simulink model "ur5_mb1"  (R2024b)
settings: Solver=VariableStepAuto  StartTime=0.0  StopTime=inf  RelTol=1e-3
values from neighbouring files (symbols this model uses):
  N = 500000    [te.m]
undefined symbols (not defined in the file or in its folder): X, Y, Z
libraries: sm_lib x89, nesl_utility x25, sldrtlib x1
(part 1 of 3)
settings Model: Creator=20844  LastModifiedBy=20844
settings ExplorerConfigSet: InternalSimMechanicsExplorerSettings="<ExplorerConfiguration><canonicalview>default</canonicalview><AnimationSetting><BasePlaybackSpeed>1.0</BasePlaybackSpeed><PlaybackSpeedFactor>1.0</PlaybackSpeedFactor></AnimationSetting><TilePanel><TileInfo><Tiles Columns=\"1\" Count=\"1\" Rows=\"1\"><Column Weight=\"1\"/><Row Weight=\"1\"/><Tile Height=\"1\" Width=\"1\" X=\"0\" Y=\"0\"/></Tiles></TileInfo><SceneInfo><SceneViewer><BGColor><R>0.60000002384185791</R><G>0.60000002384185791</G><B>0.60000002384185791</B></BGColor><Camera><DoPerspective>off</DoPerspective><Position><X>0.566882143907464497</X><Y>-0.926894596308694196</Y><Z>0.376591257371258314</Z></Position><Center><X>0.550100812264807226</X><Y>0.0723916711678013747</Y><Z>0.342748347608626824</Z></Center><Up><X>0.0212034026804047183</X><Y>0.0341957319134813531</Y><Z>0.999190205933622289</Z></Up><ViewLimDist>1</ViewLimDist><YLim>1.26913824826545474</YLim><XLim>1.85200174006144125</XLim></Camera></SceneViewer></SceneInfo></TilePanel><MechEditorPanel><Cameras/><GfxPanelCameraMap/><VideoCreator><PlaybackSpeedRatio>1.0</PlaybackSpeedRatio><FrameRate>30</FrameRate><VideoFormat>Motion JPEG AVI</VideoFormat><FrameSize>auto</FrameSize></VideoCreator></MechEditorPanel></ExplorerConfiguration>"

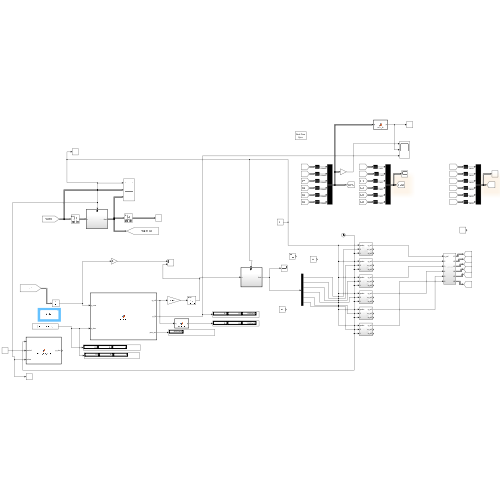
[thumbnail: Simulink's stored preview of the top-level diagram]
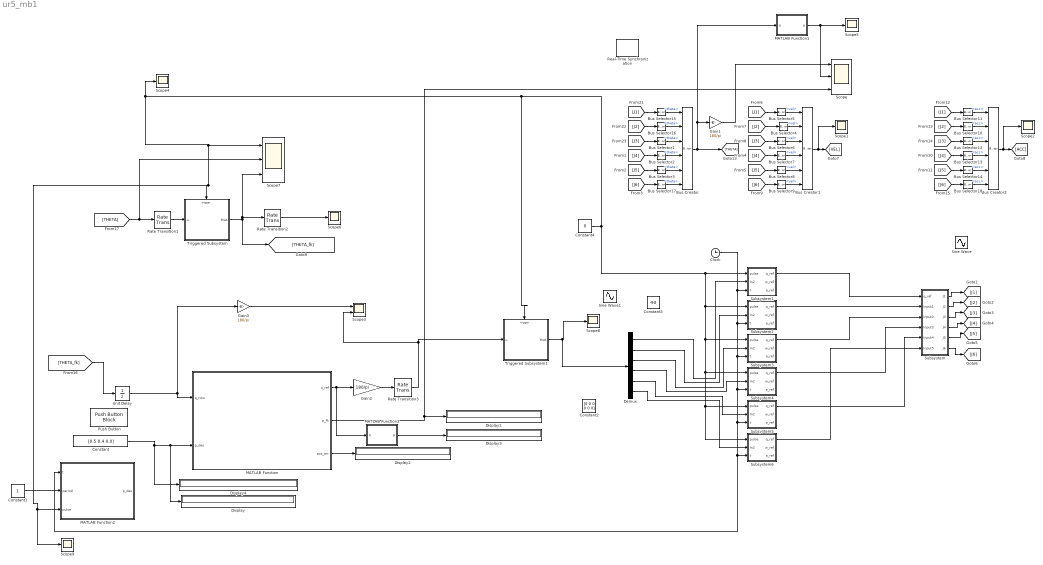
== system ur5_mb1 ==
  Bus Creator : BusCreator  Inputs=6
  Bus Creator1 : BusCreator  Inputs=6
  Bus Creator2 : BusCreator  Inputs=6
  Bus Selector{1..3,15..17} (6 alike) : BusSelector  OutputSignals=theta
  Bus Selector{10..14,18} (6 alike) : BusSelector  OutputSignals=acc
  Bus Selector{4..9} (6 alike) : BusSelector  OutputSignals=vel
  Clock : Clock
  Constant : Constant  Value=[0.5 0.4 0.0]
  Constant1 : Constant
  Constant2 : Constant  Value=[0 0 0 0 0 0]
  Constant3 : Constant  Value=-90
  Constant4 : Constant  Value=0
  Demux : Demux  Outputs=6
  Display{,1..4} (5 alike) : Display
  Gain1 : Gain  Gain=180/pi
  Gain2 : Gain  Gain=180/pi
  Gain3 : Gain  Gain=180/pi
  MATLAB Function : MATLAB Function  TreatAsAtomicUnit=on
  MATLAB Function1 : MATLAB Function  TreatAsAtomicUnit=on
  MATLAB Function2 : MATLAB Function  TreatAsAtomicUnit=on
  MATLAB Function3 : MATLAB Function  TreatAsAtomicUnit=on
  Push Button : PushButtonBlock  OnValue=2  OffValue=0.000000
  Rate Transition1 : RateTransition  OutPortSampleTime=1/100
  Rate Transition2 : RateTransition  OutPortSampleTime=1/100
  Rate Transition3 : RateTransition  OutPortSampleTime=1/100
  Real-Time Synchronization : sldrtlib/Real-Time Synchronization  SampleTime=0.001  MaxMissedTicks=inf  ShowMissedTicks=off  YieldWhenWaiting=off
  Scope : Scope  NumInputPorts=3
  Scope{1..2,4..6,8..9} (7 alike) : Scope
  Scope3 : Scope  NumInputPorts=2
  Scope7 : Scope  NumInputPorts=3
  Sine Wave : Sin  Amplitude=90  SampleTime=0
  Sine Wave1 : Sin  Amplitude=90  Frequency=5  SampleTime=0
  Subsystem : Subsystem
  Subsystem1 : Subsystem
  Subsystem2 : Subsystem
  Subsystem3 : Subsystem
  Subsystem4 : Subsystem
  Subsystem5 : Subsystem
  Subsystem6 : Subsystem
  Triggered Subsystem : Subsystem  TreatAsAtomicUnit=on
  Triggered Subsystem1 : Subsystem  TreatAsAtomicUnit=on
  Unit Delay : UnitDelay  InitialCondition=[0 0 0 0 0 0]  SampleTime=0.001  HasFrameUpgradeWarning=on
  wires:
  Subsystem/1(J1) -> [J1]
  Subsystem/2(J2) -> [J2]
  Subsystem/3(J3) -> [J3]
  Subsystem/4(J4) -> [J4]
  Subsystem/5(J5) -> [J5]
  Subsystem/6(J6) -> [J6]
  [J3] -> Bus Selector1/1
  [J2] -> Bus Selector16/1
  [J1] -> Bus Selector15/1
  Bus Selector1/1 -> Bus Creator/3  "<theta>"
  Bus Selector15/1 -> Bus Creator/1  "<theta>"
  Bus Selector16/1 -> Bus Creator/2  "<theta>"
  Bus Creator/1 -> MATLAB Function1/1(q), Gain1/1, [THETA]
  [J5] -> Bus Selector3/1
  Bus Selector3/1 -> Bus Creator/5  "<theta>"
  [J4] -> Bus Selector2/1
  Bus Selector17/1 -> Bus Creator/6  "<theta>"
  Bus Selector2/1 -> Bus Creator/4  "<theta>"
  [J6] -> Bus Selector17/1
  [J6] -> Bus Selector9/1
  Bus Selector7/1 -> Bus Creator1/4  "<vel>"
  Bus Selector9/1 -> Bus Creator1/6  "<vel>"
  [J4] -> Bus Selector7/1
  Bus Selector8/1 -> Bus Creator1/5  "<vel>"
  [J5] -> Bus Selector8/1
  Bus Creator1/1 -> Scope1/1, [VEL]
  Bus Selector4/1 -> Bus Creator1/2  "<vel>"
  Bus Selector5/1 -> Bus Creator1/1  "<vel>"
  Bus Selector6/1 -> Bus Creator1/3  "<vel>"
  [J1] -> Bus Selector5/1
  [J2] -> Bus Selector4/1
  [J3] -> Bus Selector6/1
  [J3] -> Bus Selector12/1
  [J2] -> Bus Selector10/1
  [J1] -> Bus Selector11/1
  Bus Selector12/1 -> Bus Creator2/3  "<acc>"
  Bus Selector11/1 -> Bus Creator2/1  "<acc>"
  Bus Selector10/1 -> Bus Creator2/2  "<acc>"
  [J5] -> Bus Selector14/1
  Bus Selector14/1 -> Bus Creator2/5  "<acc>"
  [J4] -> Bus Selector13/1
  Bus Selector18/1 -> Bus Creator2/6  "<acc>"
  Bus Selector13/1 -> Bus Creator2/4  "<acc>"
  [J6] -> Bus Selector18/1
  Bus Creator2/1 -> Scope2/1, [ACC]
  Gain1/1 -> Scope/1
  MATLAB Function1/1(p) -> Scope/2, Scope5/1
  Constant4/1 -> Subsystem6/1(pulse), Subsystem5/1(pulse), Subsystem4/1(pulse), Subsystem3/1(pulse), Subsystem2/1(pulse), Subsystem1/1(pulse), Triggered Subsystem1/Trigger, Scope4/1, Scope9/1, MATLAB Function2/3(pulse), Triggered Subsystem/Trigger, Scope7/1
  MATLAB Function/2(p_fk) -> Scope/3, Display1/1
  [THETA_fk] -> Unit Delay/1
  Rate Transition3/1 -> Triggered Subsystem1/1(u), Scope3/2
  Constant/1 -> Display4/1, Display/1, MATLAB Function/2(p_des)
  [THETA] -> Rate Transition1/1, Scope7/2
  Triggered Subsystem/1(thet) -> Scope7/3, Rate Transition2/1, [THETA_fk]
  Rate Transition2/1 -> Scope6/1
  Rate Transition1/1 -> Triggered Subsystem/1(u)
  MATLAB Function/1(q_ref) -> MATLAB Function3/1(q), Gain2/1
  Gain3/1 -> Scope3/1
  Subsystem1/1(q_ref) -> Subsystem/1(q_ref)
  Clock/1 -> MATLAB Function2/1(t), Subsystem6/3(t), Subsystem5/3(t), Subsystem4/3(t), Subsystem3/3(t), Subsystem2/3(t), Subsystem1/3(t)
  Subsystem2/1(q_ref) -> Subsystem/2(Input1)
  Subsystem3/1(q_ref) -> Subsystem/3(Input2)
  Subsystem4/1(q_ref) -> Subsystem/4(Input3)
  Subsystem5/1(q_ref) -> Subsystem/5(Input4)
  Subsystem6/1(q_ref) -> Subsystem/6(Input5)
  Demux/1 -> Subsystem1/2(In2)
  Demux/2 -> Subsystem2/2(In2)
  Demux/3 -> Subsystem3/2(In2)
  Demux/4 -> Subsystem4/2(In2)
  Demux/5 -> Subsystem5/2(In2)
  Demux/6 -> Subsystem6/2(In2)
  Gain2/1 -> Rate Transition3/1
  Triggered Subsystem1/1(thet) -> Demux/1, Scope8/1
  Unit Delay/1 -> Gain3/1, MATLAB Function/1(q_now)
  Constant1/1 -> MATLAB Function2/2(period)
  MATLAB Function/3(pos_err) -> Display2/1
  MATLAB Function3/1(p) -> Display3/1

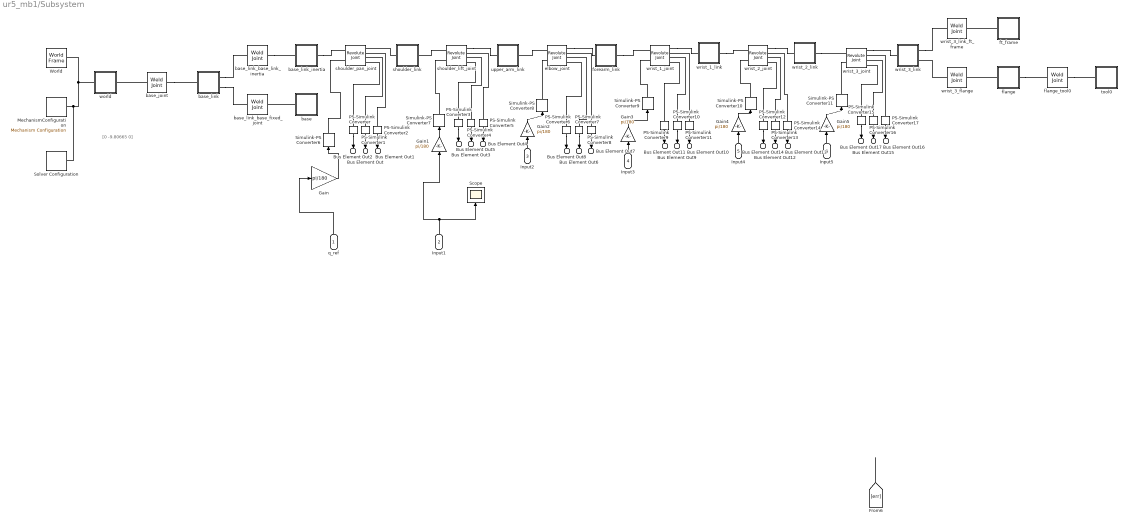
== system ur5_mb1/Subsystem ==
  note: [0 -9.80665 0]
  q_ref : Inport
  Input1 : Inport  Port=2
  Input2 : Inport  Port=3
  Input3 : Inport  Port=4
  Input4 : Inport  Port=5
  Input5 : Inport  Port=6
  Gain{,1..5} (6 alike) : Gain  Gain=pi/180
  MechanismConfiguration : sm_lib/Utilities/Mechanism Configuration  UniformGravity=Constant  GravityVector=[0 0 -9.80665]  GravityVectorUnits=m/s^2  LinearizationDelta=0.001  JointModeTransitionNonlinearIterations=2
  PS-Simulink Converter{,1..17} (18 alike) : nesl_utility/PS-Simulink Converter  PhysicalDomain=network_engine_domain  SubClassName=ps_output  LeftPortType=input  RightPortType=output  PseudoPeriodic=off  Frequencies=[]  VectorFormat=inherit  Unit=inherit  AffineConversion=off
  Scope : Scope
  Simulink-PS Converter{6..11} (6 alike) : nesl_utility/Simulink-PS Converter  PhysicalDomain=network_engine_domain  SubClassName=ps_input  LeftPortType=input  RightPortType=output  PseudoPeriodic=off  Frequencies=[]  NoiseDistribution=none  NoiseParameters=[]  Unit=rad  AffineConversion=off  FilteringAndDerivatives=filter  SimscapeFilterOrder=2  InputFilterTimeConstant=0.001  UdotUserProvided=0
  Solver Configuration : nesl_utility/Solver Configuration  PhysicalDomain=network_engine_domain  SubClassName=solver  LeftPortType=input  RightPortType=generic  Tones=[]  Harmonics=[]  SimulateNoise=off  Profile=off  UseLocalSampling=off  EnableSwitchedLinearOptims=on  FrequencyDomain=off  UseCCode=off  RelTol=0.001  AbsTol=0.001  MinStep=1e-09  ToWorkspace=off  RevertToSquareIcSolve=off  NumHomotopyIterations=100  PhasorMode=off  PhasorModeNumHarmonics=1  ConsistencySolver=NEWTON_XTOL_AFTER_FTOL  IndexReductionMethod=DerivativeReplacement  DoDC=off  ResidualTolerance=1e-09  ConsistencyTolSource=GLOBAL  ConsistencyAbsTol=0.001  ConsistencyRelTol=0.001  ConsistencyTolFactor=0.001  UseLocalSolver=off  LocalSolverChoice=NE_BACKWARD_EULER_ADVANCER  ResolveIndetEquations=on  FunctionEvalNumThread=1  LocalSolverSampleTime=0.001  DoFixedCost=off  MaxNonlinIter=3  MaxModeIter=2  ComputeImpulses=off  ImpulseIterations=2  LinearAlgebra=auto  LinearAlgebraNumThread=0  EquationFormulation=NE_TIME_EF  DelaysMemoryBudget=1024  AutomaticFiltering=on  FilteringTimeConstant=0.001  PartitionStorageMethod=AS_NEEDED  PartitionMemoryBudget=1024  PartitionMethod=ROBUST  MultibodyUseLocalSolver=off  MultibodyLocalSolverChoice=ODE1  MultibodyLocalSolverSampleTime=0.001
  World : sm_lib/Frames and Transforms/World Frame
  base : Subsystem
  base_joint : sm_lib/Joints/Weld Joint  JointMode=Normal  CompositeWrenchDir=FollowerOnBase  CompositeWrenchFrame=BaseFrame  SenseConstraintForce=off  SenseConstraintTorque=off  SenseTotalForce=off  SenseTotalTorque=off
  base_link : Subsystem
  base_link_base_fixed_joint : sm_lib/Joints/Weld Joint  JointMode=Normal  CompositeWrenchDir=FollowerOnBase  CompositeWrenchFrame=BaseFrame  SenseConstraintForce=off  SenseConstraintTorque=off  SenseTotalForce=off  SenseTotalTorque=off
  base_link_base_link_inertia : sm_lib/Joints/Weld Joint  JointMode=Normal  CompositeWrenchDir=FollowerOnBase  CompositeWrenchFrame=BaseFrame  SenseConstraintForce=off  SenseConstraintTorque=off  SenseTotalForce=off  SenseTotalTorque=off
  base_link_inertia : Subsystem
  elbow_joint : sm_lib/Joints/Revolute Joint  JointMode=Normal  CompositeWrenchDir=FollowerOnBase  CompositeWrenchFrame=BaseFrame  SenseConstraintForce=off  SenseConstraintTorque=off  SenseTotalForce=off  SenseTotalTorque=off  PositionTargetSpecify=on  PositionTargetPriority=High  PositionTargetValue=0  PositionTargetValueUnits=rad  VelocityTargetSpecify=off  VelocityTargetPriority=High  VelocityTargetValue=0  VelocityTargetValueUnits=deg/s  EquilibriumPosition=0  EquilibriumPositionUnits=deg  SpringStiffness=0  SpringStiffnessUnits=N*m/deg  DampingCoefficient=0.0  DampingCoefficientUnits=kg*m^2/(rad*s)  LowerLimitSpecify=on  LowerLimitBound=-3.141592653589793  LowerLimitBoundUnits=rad  LowerLimitStiffness=1e4  LowerLimitStiffnessUnits=N*m/deg  LowerLimitDamping=10  LowerLimitDampingUnits=N*m/(deg/s)  LowerLimitTransitionRegionWidth=0.1  LowerLimitTransitionRegionWidthUnits=deg  UpperLimitSpecify=on  UpperLimitBound=3.141592653589793  UpperLimitBoundUnits=rad  UpperLimitStiffness=1e4  UpperLimitStiffnessUnits=N*m/deg  UpperLimitDamping=10  UpperLimitDampingUnits=N*m/(deg/s)  UpperLimitTransitionRegionWidth=0.1  UpperLimitTransitionRegionWidthUnits=deg  TorqueActuationMode=ComputedTorque  MotionActuationMode=InputMotion  SensePosition=on  SenseVelocity=on  SenseAcceleration=on  SenseTorqueForce=off  SenseLowerLimitTorqueForce=off  SenseUpperLimitTorqueForce=off
  flange : Subsystem
  flange_tool0 : sm_lib/Joints/Weld Joint  JointMode=Normal  CompositeWrenchDir=FollowerOnBase  CompositeWrenchFrame=BaseFrame  SenseConstraintForce=off  SenseConstraintTorque=off  SenseTotalForce=off  SenseTotalTorque=off
  forearm_link : Subsystem
  ft_frame : Subsystem
  shoulder_lift_joint : sm_lib/Joints/Revolute Joint  JointMode=Normal  CompositeWrenchDir=FollowerOnBase  CompositeWrenchFrame=BaseFrame  SenseConstraintForce=off  SenseConstraintTorque=off  SenseTotalForce=off  SenseTotalTorque=off  PositionTargetSpecify=on  PositionTargetPriority=High  PositionTargetValue=0  PositionTargetValueUnits=rad  VelocityTargetSpecify=off  VelocityTargetPriority=High  VelocityTargetValue=0  VelocityTargetValueUnits=deg/s  EquilibriumPosition=0  EquilibriumPositionUnits=deg  SpringStiffness=0  SpringStiffnessUnits=N*m/deg  DampingCoefficient=2.0  DampingCoefficientUnits=kg*m^2/(rad*s)  LowerLimitSpecify=on  LowerLimitBound=-6.283185307179586  LowerLimitBoundUnits=rad  LowerLimitStiffness=1e4  LowerLimitStiffnessUnits=N*m/deg  LowerLimitDamping=10  LowerLimitDampingUnits=N*m/(deg/s)  LowerLimitTransitionRegionWidth=0.1  LowerLimitTransitionRegionWidthUnits=deg  UpperLimitSpecify=on  UpperLimitBound=6.283185307179586  UpperLimitBoundUnits=rad  UpperLimitStiffness=1e4  UpperLimitStiffnessUnits=N*m/deg  UpperLimitDamping=10  UpperLimitDampingUnits=N*m/(deg/s)  UpperLimitTransitionRegionWidth=0.1  UpperLimitTransitionRegionWidthUnits=deg  TorqueActuationMode=ComputedTorque  MotionActuationMode=InputMotion  SensePosition=on  SenseVelocity=on  SenseAcceleration=on  SenseTorqueForce=off  SenseLowerLimitTorqueForce=off  SenseUpperLimitTorqueForce=off
  shoulder_link : Subsystem
  shoulder_pan_joint : sm_lib/Joints/Revolute Joint  JointMode=Normal  CompositeWrenchDir=FollowerOnBase  CompositeWrenchFrame=BaseFrame  SenseConstraintForce=off  SenseConstraintTorque=off  SenseTotalForce=off  SenseTotalTorque=off  PositionTargetSpecify=on  PositionTargetPriority=High  PositionTargetValue=0  PositionTargetValueUnits=rad  VelocityTargetSpecify=off  VelocityTargetPriority=High  VelocityTargetValue=0  VelocityTargetValueUnits=deg/s  EquilibriumPosition=0  EquilibriumPositionUnits=deg  SpringStiffness=0  SpringStiffnessUnits=N*m/deg  DampingCoefficient=0.0  DampingCoefficientUnits=kg*m^2/(rad*s)  LowerLimitSpecify=on  LowerLimitBound=-6.283185307179586  LowerLimitBoundUnits=rad  LowerLimitStiffness=1e4  LowerLimitStiffnessUnits=N*m/deg  LowerLimitDamping=10  LowerLimitDampingUnits=N*m/(deg/s)  LowerLimitTransitionRegionWidth=0.1  LowerLimitTransitionRegionWidthUnits=deg  UpperLimitSpecify=on  UpperLimitBound=6.283185307179586  UpperLimitBoundUnits=rad  UpperLimitStiffness=1e4  UpperLimitStiffnessUnits=N*m/deg  UpperLimitDamping=10  UpperLimitDampingUnits=N*m/(deg/s)  UpperLimitTransitionRegionWidth=0.1  UpperLimitTransitionRegionWidthUnits=deg  TorqueActuationMode=ComputedTorque  MotionActuationMode=InputMotion  SensePosition=on  SenseVelocity=on  SenseAcceleration=on  SenseTorqueForce=off  SenseLowerLimitTorqueForce=off  SenseUpperLimitTorqueForce=off
  tool0 : Subsystem
  upper_arm_link : Subsystem
  world : Subsystem
  wrist_1_joint : sm_lib/Joints/Revolute Joint  JointMode=Normal  CompositeWrenchDir=FollowerOnBase  CompositeWrenchFrame=BaseFrame  SenseConstraintForce=off  SenseConstraintTorque=off  SenseTotalForce=off  SenseTotalTorque=off  PositionTargetSpecify=on  PositionTargetPriority=High  PositionTargetValue=0  PositionTargetValueUnits=rad  VelocityTargetSpecify=off  VelocityTargetPriority=High  VelocityTargetValue=0  VelocityTargetValueUnits=deg/s  EquilibriumPosition=0  EquilibriumPositionUnits=deg  SpringStiffness=0  SpringStiffnessUnits=N*m/deg  DampingCoefficient=0.0  DampingCoefficientUnits=kg*m^2/(rad*s)  LowerLimitSpecify=on  LowerLimitBound=-6.283185307179586  LowerLimitBoundUnits=rad  LowerLimitStiffness=1e4  LowerLimitStiffnessUnits=N*m/deg  LowerLimitDamping=10  LowerLimitDampingUnits=N*m/(deg/s)  LowerLimitTransitionRegionWidth=0.1  LowerLimitTransitionRegionWidthUnits=deg  UpperLimitSpecify=on  UpperLimitBound=6.283185307179586  UpperLimitBoundUnits=rad  UpperLimitStiffness=1e4  UpperLimitStiffnessUnits=N*m/deg  UpperLimitDamping=10  UpperLimitDampingUnits=N*m/(deg/s)  UpperLimitTransitionRegionWidth=0.1  UpperLimitTransitionRegionWidthUnits=deg  TorqueActuationMode=ComputedTorque  MotionActuationMode=InputMotion  SensePosition=on  SenseVelocity=on  SenseAcceleration=on  SenseTorqueForce=off  SenseLowerLimitTorqueForce=off  SenseUpperLimitTorqueForce=off
  wrist_1_link : Subsystem
  wrist_2_joint : sm_lib/Joints/Revolute Joint  JointMode=Normal  CompositeWrenchDir=FollowerOnBase  CompositeWrenchFrame=BaseFrame  SenseConstraintForce=off  SenseConstraintTorque=off  SenseTotalForce=off  SenseTotalTorque=off  PositionTargetSpecify=on  PositionTargetPriority=High  PositionTargetValue=0  PositionTargetValueUnits=rad  VelocityTargetSpecify=off  VelocityTargetPriority=High  VelocityTargetValue=0  VelocityTargetValueUnits=deg/s  EquilibriumPosition=0  EquilibriumPositionUnits=deg  SpringStiffness=0  SpringStiffnessUnits=N*m/deg  DampingCoefficient=0.0  DampingCoefficientUnits=kg*m^2/(rad*s)  LowerLimitSpecify=on  LowerLimitBound=-6.283185307179586  LowerLimitBoundUnits=rad  LowerLimitStiffness=1e4  LowerLimitStiffnessUnits=N*m/deg  LowerLimitDamping=10  LowerLimitDampingUnits=N*m/(deg/s)  LowerLimitTransitionRegionWidth=0.1  LowerLimitTransitionRegionWidthUnits=deg  UpperLimitSpecify=on  UpperLimitBound=6.283185307179586  UpperLimitBoundUnits=rad  UpperLimitStiffness=1e4  UpperLimitStiffnessUnits=N*m/deg  UpperLimitDamping=10  UpperLimitDampingUnits=N*m/(deg/s)  UpperLimitTransitionRegionWidth=0.1  UpperLimitTransitionRegionWidthUnits=deg  TorqueActuationMode=ComputedTorque  MotionActuationMode=InputMotion  SensePosition=on  SenseVelocity=on  SenseAcceleration=on  SenseTorqueForce=off  SenseLowerLimitTorqueForce=off  SenseUpperLimitTorqueForce=off
  wrist_2_link : Subsystem
  wrist_3_flange : sm_lib/Joints/Weld Joint  JointMode=Normal  CompositeWrenchDir=FollowerOnBase  CompositeWrenchFrame=BaseFrame  SenseConstraintForce=off  SenseConstraintTorque=off  SenseTotalForce=off  SenseTotalTorque=off
  wrist_3_joint : sm_lib/Joints/Revolute Joint  JointMode=Normal  CompositeWrenchDir=FollowerOnBase  CompositeWrenchFrame=BaseFrame  SenseConstraintForce=off  SenseConstraintTorque=off  SenseTotalForce=off  SenseTotalTorque=off  PositionTargetSpecify=on  PositionTargetPriority=High  PositionTargetValue=0  PositionTargetValueUnits=rad  VelocityTargetSpecify=off  VelocityTargetPriority=High  VelocityTargetValue=0  VelocityTargetValueUnits=deg/s  EquilibriumPosition=0  EquilibriumPositionUnits=deg  SpringStiffness=0  SpringStiffnessUnits=N*m/deg  DampingCoefficient=0.0  DampingCoefficientUnits=kg*m^2/(rad*s)  LowerLimitSpecify=on  LowerLimitBound=-6.283185307179586  LowerLimitBoundUnits=rad  LowerLimitStiffness=1e4  LowerLimitStiffnessUnits=N*m/deg  LowerLimitDamping=10  LowerLimitDampingUnits=N*m/(deg/s)  LowerLimitTransitionRegionWidth=0.1  LowerLimitTransitionRegionWidthUnits=deg  UpperLimitSpecify=on  UpperLimitBound=6.283185307179586  UpperLimitBoundUnits=rad  UpperLimitStiffness=1e4  UpperLimitStiffnessUnits=N*m/deg  UpperLimitDamping=10  UpperLimitDampingUnits=N*m/(deg/s)  UpperLimitTransitionRegionWidth=0.1  UpperLimitTransitionRegionWidthUnits=deg  TorqueActuationMode=ComputedTorque  MotionActuationMode=InputMotion  SensePosition=on  SenseVelocity=on  SenseAcceleration=on  SenseTorqueForce=off  SenseLowerLimitTorqueForce=off  SenseUpperLimitTorqueForce=off
  wrist_3_link : Subsystem
  wrist_3_link_ft_frame : sm_lib/Joints/Weld Joint  JointMode=Normal  CompositeWrenchDir=FollowerOnBase  CompositeWrenchFrame=BaseFrame  SenseConstraintForce=off  SenseConstraintTorque=off  SenseTotalForce=off  SenseTotalTorque=off
  Bus Element Out : Outport  PortName=J1  Element=vel
  Bus Element Out1 : Outport  PortName=J1  Element=theta
  Bus Element Out2 : Outport  PortName=J1  Element=acc
  Bus Element Out3 : Outport  Port=2  PortName=J2  Element=vel
  Bus Element Out4 : Outport  Port=2  PortName=J2  Element=theta
  Bus Element Out5 : Outport  Port=2  PortName=J2  Element=acc
  Bus Element Out6 : Outport  Port=3  PortName=J3  Element=vel
  Bus Element Out7 : Outport  Port=3  PortName=J3  Element=theta
  Bus Element Out8 : Outport  Port=3  PortName=J3  Element=acc
  Bus Element Out9 : Outport  Port=4  PortName=J4  Element=vel
  Bus Element Out10 : Outport  Port=4  PortName=J4  Element=theta
  Bus Element Out11 : Outport  Port=4  PortName=J4  Element=acc
  Bus Element Out12 : Outport  Port=5  PortName=J5  Element=vel
  Bus Element Out13 : Outport  Port=5  PortName=J5  Element=theta
  Bus Element Out14 : Outport  Port=5  PortName=J5  Element=acc
  Bus Element Out15 : Outport  Port=6  PortName=J6  Element=vel
  Bus Element Out16 : Outport  Port=6  PortName=J6  Element=theta
  Bus Element Out17 : Outport  Port=6  PortName=J6  Element=acc
  wires:
  q_ref/1 -> Gain/1
  Input2/1 -> Gain2/1
  Input3/1 -> Gain3/1
  Input4/1 -> Gain4/1
  Input5/1 -> Gain5/1
  PS-Simulink Converter/1 -> Bus Element Out2/1
  PS-Simulink Converter1/1 -> Bus Element Out/1
  PS-Simulink Converter2/1 -> Bus Element Out1/1
  PS-Simulink Converter3/1 -> Bus Element Out5/1
  PS-Simulink Converter4/1 -> Bus Element Out3/1
  PS-Simulink Converter5/1 -> Bus Element Out4/1
  PS-Simulink Converter6/1 -> Bus Element Out8/1
  PS-Simulink Converter7/1 -> Bus Element Out6/1
  PS-Simulink Converter8/1 -> Bus Element Out7/1
  PS-Simulink Converter9/1 -> Bus Element Out11/1
  PS-Simulink Converter10/1 -> Bus Element Out9/1
  PS-Simulink Converter11/1 -> Bus Element Out10/1
  PS-Simulink Converter12/1 -> Bus Element Out14/1
  PS-Simulink Converter13/1 -> Bus Element Out12/1
  PS-Simulink Converter14/1 -> Bus Element Out13/1
  PS-Simulink Converter15/1 -> Bus Element Out17/1
  PS-Simulink Converter16/1 -> Bus Element Out15/1
  PS-Simulink Converter17/1 -> Bus Element Out16/1
  Input1/1 -> Gain1/1, Scope/1
  Gain/1 -> Simulink-PS Converter6/1
  Gain1/1 -> Simulink-PS Converter7/1
  Gain2/1 -> Simulink-PS Converter8/1
  Gain5/1 -> Simulink-PS Converter11/1
  Gain4/1 -> Simulink-PS Converter10/1
  Gain3/1 -> Simulink-PS Converter9/1
  [err] -> ?
  connections:
  shoulder_link/LConn1 -- shoulder_pan_joint/RConn1
  ft_frame/LConn1 -- wrist_3_link_ft_frame/RConn1
  World/RConn1 -- MechanismConfiguration/RConn1 -- Solver Configuration/RConn1 -- world/LConn1
  base_link/RConn2 -- base_link_base_fixed_joint/LConn1
  wrist_2_joint/RConn1 -- wrist_2_link/LConn1
  elbow_joint/LConn1 -- upper_arm_link/RConn1
  base_joint/LConn1 -- world/RConn1
  base/LConn1 -- base_link_base_fixed_joint/RConn1
  flange_tool0/RConn1 -- tool0/LConn1
  shoulder_lift_joint/LConn1 -- shoulder_link/RConn1
  base_link/RConn1 -- base_link_base_link_inertia/LConn1
  forearm_link/RConn1 -- wrist_1_joint/LConn1
  flange/LConn1 -- wrist_3_flange/RConn1
  wrist_1_link/RConn1 -- wrist_2_joint/LConn1
  elbow_joint/RConn1 -- forearm_link/LConn1
  wrist_3_flange/LConn1 -- wrist_3_link/RConn2
  flange/RConn1 -- flange_tool0/LConn1
  base_joint/RConn1 -- base_link/LConn1
  wrist_1_joint/RConn1 -- wrist_1_link/LConn1
  wrist_3_joint/RConn1 -- wrist_3_link/LConn1
  wrist_3_link/RConn1 -- wrist_3_link_ft_frame/LConn1
  base_link_inertia/RConn1 -- shoulder_pan_joint/LConn1
  base_link_base_link_inertia/RConn1 -- base_link_inertia/LConn1
  wrist_2_link/RConn1 -- wrist_3_joint/LConn1
  shoulder_lift_joint/RConn1 -- upper_arm_link/LConn1
  PS-Simulink Converter2/LConn1 -- shoulder_pan_joint/RConn2
  PS-Simulink Converter1/LConn1 -- shoulder_pan_joint/RConn3
  PS-Simulink Converter/LConn1 -- shoulder_pan_joint/RConn4
  PS-Simulink Converter5/LConn1 -- shoulder_lift_joint/RConn2
  PS-Simulink Converter4/LConn1 -- shoulder_lift_joint/RConn3
  PS-Simulink Converter3/LConn1 -- shoulder_lift_joint/RConn4
  PS-Simulink Converter8/LConn1 -- elbow_joint/RConn2
  PS-Simulink Converter7/LConn1 -- elbow_joint/RConn3
  PS-Simulink Converter6/LConn1 -- elbow_joint/RConn4
  PS-Simulink Converter11/LConn1 -- wrist_1_joint/RConn2
  PS-Simulink Converter10/LConn1 -- wrist_1_joint/RConn3
  PS-Simulink Converter9/LConn1 -- wrist_1_joint/RConn4
  PS-Simulink Converter14/LConn1 -- wrist_2_joint/RConn2
  PS-Simulink Converter13/LConn1 -- wrist_2_joint/RConn3
  PS-Simulink Converter12/LConn1 -- wrist_2_joint/RConn4
  PS-Simulink Converter17/LConn1 -- wrist_3_joint/RConn2
  PS-Simulink Converter16/LConn1 -- wrist_3_joint/RConn3
  PS-Simulink Converter15/LConn1 -- wrist_3_joint/RConn4
  Simulink-PS Converter6/RConn1 -- shoulder_pan_joint/LConn2
  Simulink-PS Converter7/RConn1 -- shoulder_lift_joint/LConn2
  Simulink-PS Converter8/RConn1 -- elbow_joint/LConn2
  Simulink-PS Converter9/RConn1 -- wrist_1_joint/LConn2
  Simulink-PS Converter10/RConn1 -- wrist_2_joint/LConn2
  Simulink-PS Converter11/RConn1 -- wrist_3_joint/LConn2

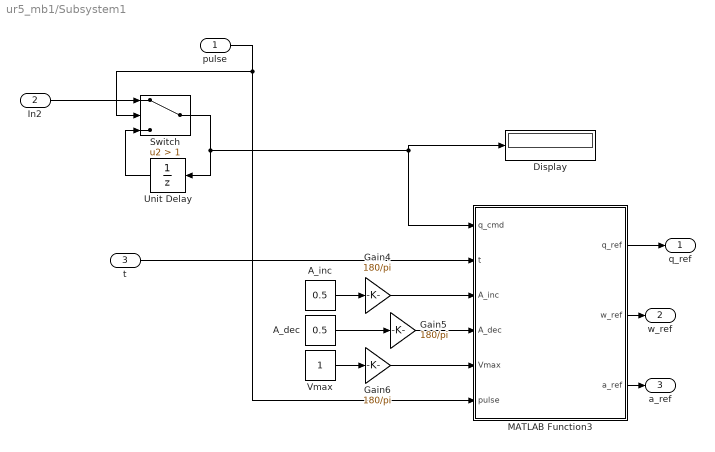
== system ur5_mb1/Subsystem1 ==
  pulse : Inport
  In2 : Inport  Port=2
  t : Inport  Port=3
  A_dec : Constant  Value=0.5
  "A_inc " : Constant  Value=0.5
  Display : Display
  Gain4 : Gain  Gain=180/pi
  Gain5 : Gain  Gain=180/pi
  Gain6 : Gain  Gain=180/pi
  MATLAB Function3 : MATLAB Function  TreatAsAtomicUnit=on
  Switch : Switch  Criteria=u2 > Threshold  Threshold=1  SaturateOnIntegerOverflow=off  InputSameDT=off
  Unit Delay : UnitDelay  SampleTime=-1  HasFrameUpgradeWarning=on
  "Vmax  " : Constant
  q_ref : Outport
  w_ref : Outport  Port=2
  a_ref : Outport  Port=3
  wires:
  MATLAB Function3/2(w_ref) -> w_ref/1
  A_dec/1 -> Gain5/1
  Switch/1 -> Unit Delay/1, Display/1, MATLAB Function3/1(q_cmd)
  Gain6/1 -> MATLAB Function3/5(Vmax)
  Gain4/1 -> MATLAB Function3/3(A_inc)
  pulse/1 -> MATLAB Function3/6(pulse), Switch/2
  "A_inc "/1 -> Gain4/1
  Gain5/1 -> MATLAB Function3/4(A_dec)
  "Vmax  "/1 -> Gain6/1
  Unit Delay/1 -> Switch/3
  t/1 -> MATLAB Function3/2(t)
  MATLAB Function3/3(a_ref) -> a_ref/1
  In2/1 -> Switch/1
  MATLAB Function3/1(q_ref) -> q_ref/1

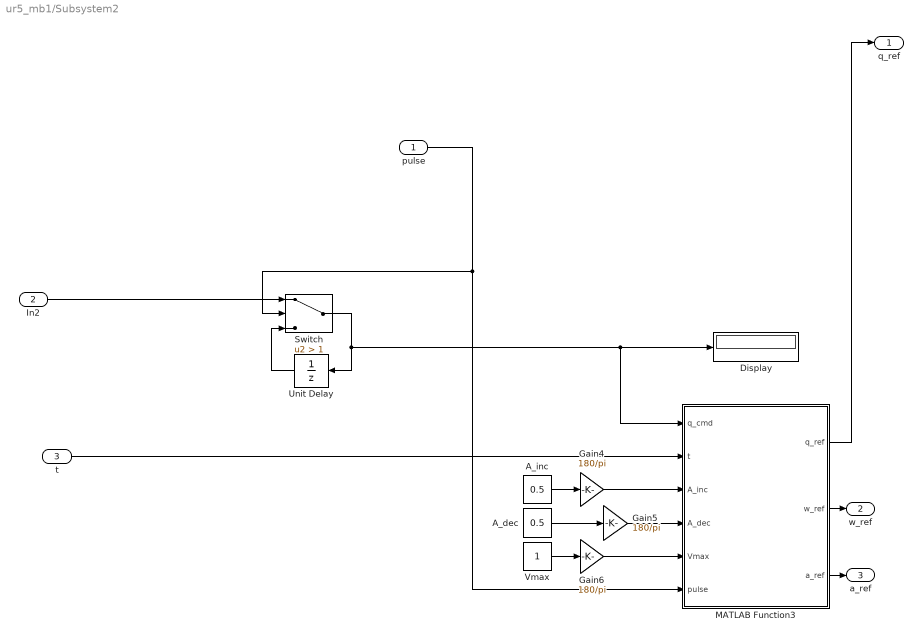
== system ur5_mb1/Subsystem2 ==
  pulse : Inport
  In2 : Inport  Port=2
  t : Inport  Port=3
  A_dec : Constant  Value=0.5
  "A_inc " : Constant  Value=0.5
  Display : Display
  Gain4 : Gain  Gain=180/pi
  Gain5 : Gain  Gain=180/pi
  Gain6 : Gain  Gain=180/pi
  MATLAB Function3 : MATLAB Function  TreatAsAtomicUnit=on
  Switch : Switch  Criteria=u2 > Threshold  Threshold=1  SaturateOnIntegerOverflow=off  InputSameDT=off
  Unit Delay : UnitDelay  SampleTime=-1  HasFrameUpgradeWarning=on
  "Vmax  " : Constant
  q_ref : Outport
  w_ref : Outport  Port=2
  a_ref : Outport  Port=3
  wires:
  MATLAB Function3/1(q_ref) -> q_ref/1
  In2/1 -> Switch/1
  MATLAB Function3/3(a_ref) -> a_ref/1
  t/1 -> MATLAB Function3/2(t)
  Unit Delay/1 -> Switch/3
  "Vmax  "/1 -> Gain6/1
  Gain5/1 -> MATLAB Function3/4(A_dec)
  "A_inc "/1 -> Gain4/1
  pulse/1 -> Switch/2, MATLAB Function3/6(pulse)
  Gain4/1 -> MATLAB Function3/3(A_inc)
  Gain6/1 -> MATLAB Function3/5(Vmax)
  Switch/1 -> Display/1, MATLAB Function3/1(q_cmd), Unit Delay/1
  A_dec/1 -> Gain5/1
  MATLAB Function3/2(w_ref) -> w_ref/1

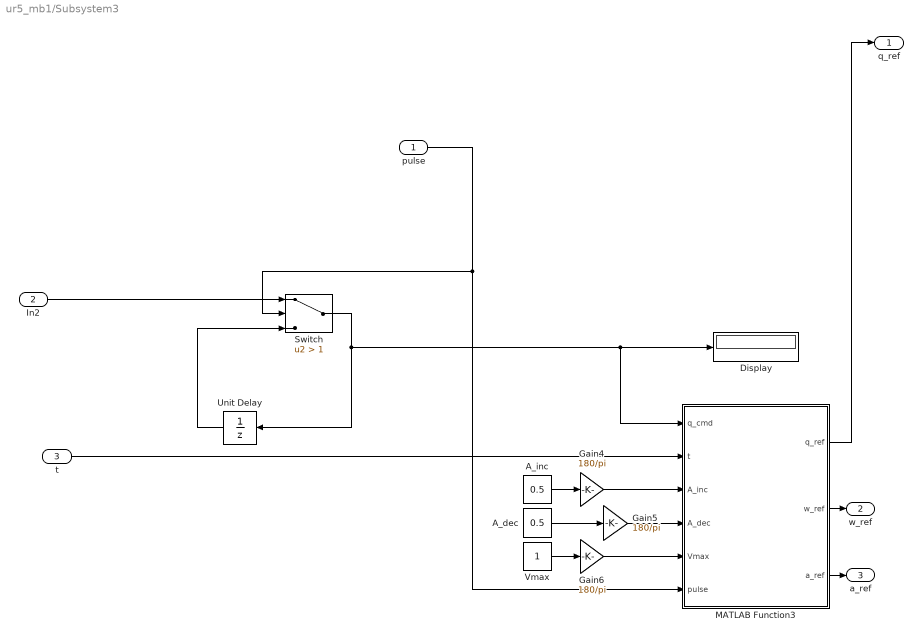
== system ur5_mb1/Subsystem3 ==
  pulse : Inport
  In2 : Inport  Port=2
  t : Inport  Port=3
  A_dec : Constant  Value=0.5
  "A_inc " : Constant  Value=0.5
  Display : Display
  Gain4 : Gain  Gain=180/pi
  Gain5 : Gain  Gain=180/pi
  Gain6 : Gain  Gain=180/pi
  MATLAB Function3 : MATLAB Function  TreatAsAtomicUnit=on
  Switch : Switch  Criteria=u2 > Threshold  Threshold=1  SaturateOnIntegerOverflow=off  InputSameDT=off
  Unit Delay : UnitDelay  SampleTime=-1  HasFrameUpgradeWarning=on
  "Vmax  " : Constant
  q_ref : Outport
  w_ref : Outport  Port=2
  a_ref : Outport  Port=3
  wires:
  MATLAB Function3/2(w_ref) -> w_ref/1
  A_dec/1 -> Gain5/1
  Gain6/1 -> MATLAB Function3/5(Vmax)
  Gain4/1 -> MATLAB Function3/3(A_inc)
  pulse/1 -> MATLAB Function3/6(pulse), Switch/2
  "A_inc "/1 -> Gain4/1
  Gain5/1 -> MATLAB Function3/4(A_dec)
  "Vmax  "/1 -> Gain6/1
  Unit Delay/1 -> Switch/3
  t/1 -> MATLAB Function3/2(t)
  MATLAB Function3/3(a_ref) -> a_ref/1
  In2/1 -> Switch/1
  MATLAB Function3/1(q_ref) -> q_ref/1
  Switch/1 -> Unit Delay/1, MATLAB Function3/1(q_cmd), Display/1

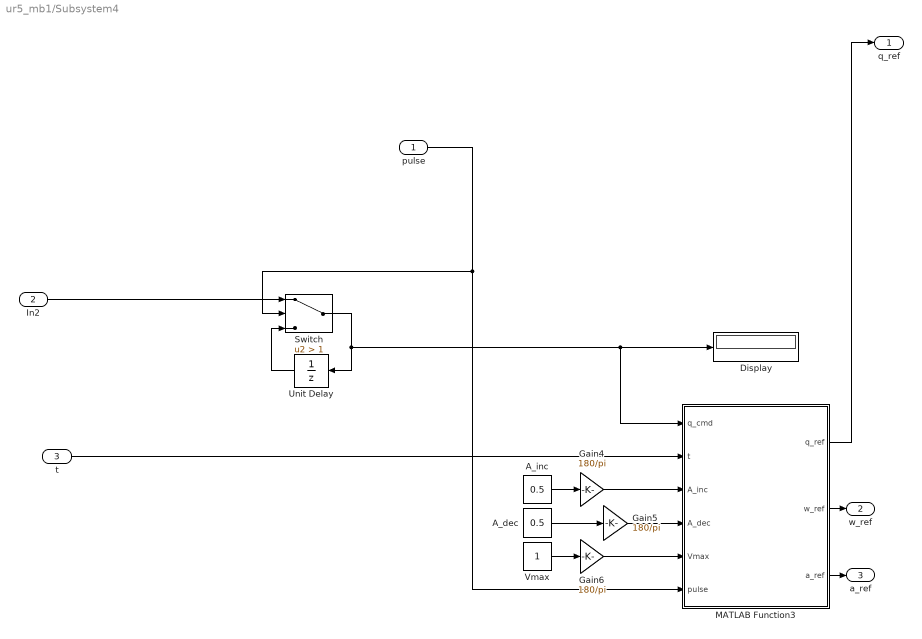
== system ur5_mb1/Subsystem4 ==
  pulse : Inport
  In2 : Inport  Port=2
  t : Inport  Port=3
  A_dec : Constant  Value=0.5
  "A_inc " : Constant  Value=0.5
  Display : Display
  Gain4 : Gain  Gain=180/pi
  Gain5 : Gain  Gain=180/pi
  Gain6 : Gain  Gain=180/pi
  MATLAB Function3 : MATLAB Function  TreatAsAtomicUnit=on
  Switch : Switch  Criteria=u2 > Threshold  Threshold=1  SaturateOnIntegerOverflow=off  InputSameDT=off
  Unit Delay : UnitDelay  SampleTime=-1  HasFrameUpgradeWarning=on
  "Vmax  " : Constant
  q_ref : Outport
  w_ref : Outport  Port=2
  a_ref : Outport  Port=3
  wires:
  MATLAB Function3/1(q_ref) -> q_ref/1
  In2/1 -> Switch/1
  MATLAB Function3/3(a_ref) -> a_ref/1
  t/1 -> MATLAB Function3/2(t)
  Unit Delay/1 -> Switch/3
  "Vmax  "/1 -> Gain6/1
  Gain5/1 -> MATLAB Function3/4(A_dec)
  "A_inc "/1 -> Gain4/1
  pulse/1 -> Switch/2, MATLAB Function3/6(pulse)
  Gain4/1 -> MATLAB Function3/3(A_inc)
  Gain6/1 -> MATLAB Function3/5(Vmax)
  Switch/1 -> Display/1, MATLAB Function3/1(q_cmd), Unit Delay/1
  A_dec/1 -> Gain5/1
  MATLAB Function3/2(w_ref) -> w_ref/1

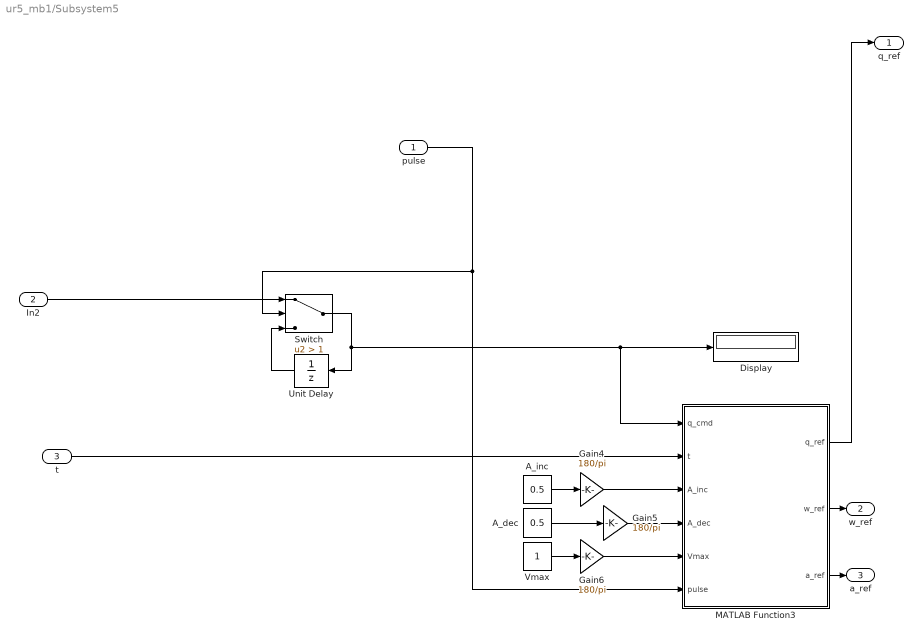
== system ur5_mb1/Subsystem5 ==
  pulse : Inport
  In2 : Inport  Port=2
  t : Inport  Port=3
  A_dec : Constant  Value=0.5
  "A_inc " : Constant  Value=0.5
  Display : Display
  Gain4 : Gain  Gain=180/pi
  Gain5 : Gain  Gain=180/pi
  Gain6 : Gain  Gain=180/pi
  MATLAB Function3 : MATLAB Function  TreatAsAtomicUnit=on
  Switch : Switch  Criteria=u2 > Threshold  Threshold=1  SaturateOnIntegerOverflow=off  InputSameDT=off
  Unit Delay : UnitDelay  SampleTime=-1  HasFrameUpgradeWarning=on
  "Vmax  " : Constant
  q_ref : Outport
  w_ref : Outport  Port=2
  a_ref : Outport  Port=3
  wires:
  MATLAB Function3/2(w_ref) -> w_ref/1
  A_dec/1 -> Gain5/1
  Switch/1 -> Unit Delay/1, MATLAB Function3/1(q_cmd), Display/1
  Gain6/1 -> MATLAB Function3/5(Vmax)
  Gain4/1 -> MATLAB Function3/3(A_inc)
  pulse/1 -> MATLAB Function3/6(pulse), Switch/2
  "A_inc "/1 -> Gain4/1
  Gain5/1 -> MATLAB Function3/4(A_dec)
  "Vmax  "/1 -> Gain6/1
  Unit Delay/1 -> Switch/3
  t/1 -> MATLAB Function3/2(t)
  MATLAB Function3/3(a_ref) -> a_ref/1
  In2/1 -> Switch/1
  MATLAB Function3/1(q_ref) -> q_ref/1

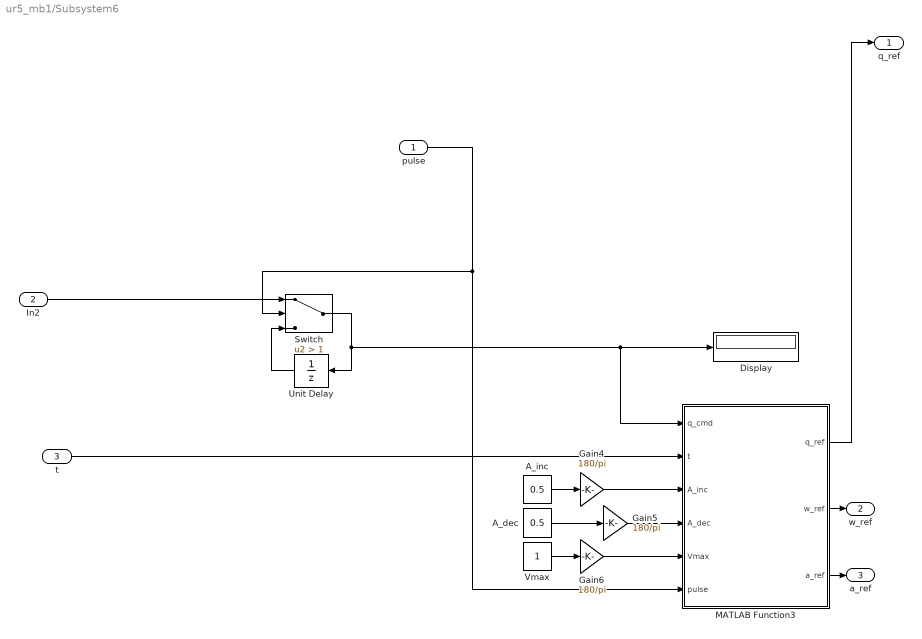
== system ur5_mb1/Subsystem6 ==
  pulse : Inport
  In2 : Inport  Port=2
  t : Inport  Port=3
  A_dec : Constant  Value=0.5
  "A_inc " : Constant  Value=0.5
  Display : Display
  Gain4 : Gain  Gain=180/pi
  Gain5 : Gain  Gain=180/pi
  Gain6 : Gain  Gain=180/pi
  MATLAB Function3 : MATLAB Function  TreatAsAtomicUnit=on
  Switch : Switch  Criteria=u2 > Threshold  Threshold=1  SaturateOnIntegerOverflow=off  InputSameDT=off
  Unit Delay : UnitDelay  SampleTime=-1  HasFrameUpgradeWarning=on
  "Vmax  " : Constant
  q_ref : Outport
  w_ref : Outport  Port=2
  a_ref : Outport  Port=3
  wires:
  MATLAB Function3/1(q_ref) -> q_ref/1
  In2/1 -> Switch/1
  MATLAB Function3/3(a_ref) -> a_ref/1
  t/1 -> MATLAB Function3/2(t)
  Unit Delay/1 -> Switch/3
  "Vmax  "/1 -> Gain6/1
  Gain5/1 -> MATLAB Function3/4(A_dec)
  "A_inc "/1 -> Gain4/1
  pulse/1 -> Switch/2, MATLAB Function3/6(pulse)
  Gain4/1 -> MATLAB Function3/3(A_inc)
  Gain6/1 -> MATLAB Function3/5(Vmax)
  Switch/1 -> Display/1, MATLAB Function3/1(q_cmd), Unit Delay/1
  A_dec/1 -> Gain5/1
  MATLAB Function3/2(w_ref) -> w_ref/1

== system ur5_mb1/Triggered Subsystem ==
  u : Inport
  Trigger : TriggerPort  VariantControl=(inherit)
  Constant : Constant  Commented=on  Value=5
  MATLAB Function : MATLAB Function  Commented=on  TreatAsAtomicUnit=on
  Sum : Sum  Commented=on  Inputs=|++
  Unit Delay : UnitDelay  Commented=on  InitialCondition=10  InputProcessing=Columns as channels (frame based)  SampleTime=-1  HasFrameUpgradeWarning=on
  thet : Outport
  wires:
  Unit Delay/1 -> Sum/1
  MATLAB Function/1(y) -> Sum/2
  Sum/1 -> Unit Delay/1
  Constant/1 -> MATLAB Function/2(data)
  u/1 -> thet/1

== system ur5_mb1/Triggered Subsystem1 ==
  u : Inport
  Trigger : TriggerPort  VariantControl=(inherit)
  Constant : Constant  Commented=on  Value=5
  MATLAB Function : MATLAB Function  Commented=on  TreatAsAtomicUnit=on
  Sum : Sum  Commented=on  Inputs=|++
  Unit Delay : UnitDelay  Commented=on  InitialCondition=10  InputProcessing=Columns as channels (frame based)  SampleTime=-1  HasFrameUpgradeWarning=on
  thet : Outport
  wires:
  Unit Delay/1 -> Sum/1
  MATLAB Function/1(y) -> Sum/2
  Sum/1 -> Unit Delay/1
  Constant/1 -> MATLAB Function/2(data)
  u/1 -> thet/1

== system ur5_mb1/Subsystem/base ==
  Inertia : sm_lib/Body Elements/Inertia  InertiaType=Custom  Mass=0  MassUnits=kg  CenterOfMass=[0, 0, 0]  CenterOfMassUnits=m  MomentsOfInertia=[0, 0, 0]  MomentsOfInertiaUnits=kg*m^2  ProductsOfInertia=[0, 0, 0]  ProductsOfInertiaUnits=kg*m^2  GraphicType=None  MarkerShape=Inertia  MarkerSize=20  GraphicVisPropType=SimpleVisualProperties  GraphicDiffuseColor=[0.5 0.5 0.5]  GraphicOpacity=1  GraphicSpecularColor=[0.5 0.5 0.5 1.0]  GraphicAmbientColor=[0.15 0.15 0.15 1.0]  GraphicEmissiveColor=[0.0 0.0 0.0 1.0]  GraphicShininess=75
  InertiaOriginTransform : sm_lib/Frames and Transforms/Rigid Transform  RotationMethod=RotationSequence  FollAlignAxisA=+X  BaseAlignAxisA=+Y  FollAlignAxisB=+Y  BaseAlignAxisB=+Z  RotationStandardAxis=+Z  RotationAngle=0  RotationAngleUnits=deg  RotationArbitraryAxis=[0 0 1]  RotationSequenceAxes=BaseAxes  RotationSequence=XYZ  RotationSequenceAngles=[0, 0, 0]  RotationSequenceAnglesUnits=rad  RotationMatrix=[1 0 0;0 1 0;0 0 1]  Quaternion=[1 0 0 0]  TranslationMethod=Cartesian  TranslationCartesianOffset=[0, 0, 0]  TranslationCartesianOffsetUnits=m  TranslationStandardAxis=+Z  TranslationStandardOffset=0  TranslationStandardOffsetUnits=m  TranslationROffset=0  TranslationROffsetUnits=m  TranslationThetaOffset=0  TranslationThetaOffsetUnits=deg  TranslationZOffset=0  TranslationZOffsetUnits=m
  ReferenceFrame : sm_lib/Frames and Transforms/Reference Frame
  F : PMIOPort  Side=Left
  connections:
  Inertia/RConn1 -- InertiaOriginTransform/RConn1
  ReferenceFrame/RConn1 -- InertiaOriginTransform/LConn1 -- F/RConn1

== system ur5_mb1/Subsystem/base_link ==
  Inertia : sm_lib/Body Elements/Inertia  InertiaType=Custom  Mass=0  MassUnits=kg  CenterOfMass=[0, 0, 0]  CenterOfMassUnits=m  MomentsOfInertia=[0, 0, 0]  MomentsOfInertiaUnits=kg*m^2  ProductsOfInertia=[0, 0, 0]  ProductsOfInertiaUnits=kg*m^2  GraphicType=None  MarkerShape=Inertia  MarkerSize=20  GraphicVisPropType=SimpleVisualProperties  GraphicDiffuseColor=[0.5 0.5 0.5]  GraphicOpacity=1  GraphicSpecularColor=[0.5 0.5 0.5 1.0]  GraphicAmbientColor=[0.15 0.15 0.15 1.0]  GraphicEmissiveColor=[0.0 0.0 0.0 1.0]  GraphicShininess=75
  InertiaOriginTransform : sm_lib/Frames and Transforms/Rigid Transform  RotationMethod=RotationSequence  FollAlignAxisA=+X  BaseAlignAxisA=+Y  FollAlignAxisB=+Y  BaseAlignAxisB=+Z  RotationStandardAxis=+Z  RotationAngle=0  RotationAngleUnits=deg  RotationArbitraryAxis=[0 0 1]  RotationSequenceAxes=BaseAxes  RotationSequence=XYZ  RotationSequenceAngles=[0, 0, 0]  RotationSequenceAnglesUnits=rad  RotationMatrix=[1 0 0;0 1 0;0 0 1]  Quaternion=[1 0 0 0]  TranslationMethod=Cartesian  TranslationCartesianOffset=[0, 0, 0]  TranslationCartesianOffsetUnits=m  TranslationStandardAxis=+Z  TranslationStandardOffset=0  TranslationStandardOffsetUnits=m  TranslationROffset=0  TranslationROffsetUnits=m  TranslationThetaOffset=0  TranslationThetaOffsetUnits=deg  TranslationZOffset=0  TranslationZOffsetUnits=m
  ReferenceFrame : sm_lib/Frames and Transforms/Reference Frame
  base_link_base_fixed_joint_OriginTransform : sm_lib/Frames and Transforms/Rigid Transform  RotationMethod=RotationSequence  FollAlignAxisA=+X  BaseAlignAxisA=+Y  FollAlignAxisB=+Y  BaseAlignAxisB=+Z  RotationStandardAxis=+Z  RotationAngle=0  RotationAngleUnits=deg  RotationArbitraryAxis=[0 0 1]  RotationSequenceAxes=BaseAxes  RotationSequence=XYZ  RotationSequenceAngles=[0, 0, 3.141592653589793]  RotationSequenceAnglesUnits=rad  RotationMatrix=[1 0 0;0 1 0;0 0 1]  Quaternion=[1 0 0 0]  TranslationMethod=Cartesian  TranslationCartesianOffset=[0, 0, 0]  TranslationCartesianOffsetUnits=m  TranslationStandardAxis=+Z  TranslationStandardOffset=0  TranslationStandardOffsetUnits=m  TranslationROffset=0  TranslationROffsetUnits=m  TranslationThetaOffset=0  TranslationThetaOffsetUnits=deg  TranslationZOffset=0  TranslationZOffsetUnits=m
  base_link_base_link_inertia_OriginTransform : sm_lib/Frames and Transforms/Rigid Transform  RotationMethod=RotationSequence  FollAlignAxisA=+X  BaseAlignAxisA=+Y  FollAlignAxisB=+Y  BaseAlignAxisB=+Z  RotationStandardAxis=+Z  RotationAngle=0  RotationAngleUnits=deg  RotationArbitraryAxis=[0 0 1]  RotationSequenceAxes=BaseAxes  RotationSequence=XYZ  RotationSequenceAngles=[0, 0, 3.141592653589793]  RotationSequenceAnglesUnits=rad  RotationMatrix=[1 0 0;0 1 0;0 0 1]  Quaternion=[1 0 0 0]  TranslationMethod=Cartesian  TranslationCartesianOffset=[0, 0, 0]  TranslationCartesianOffsetUnits=m  TranslationStandardAxis=+Z  TranslationStandardOffset=0  TranslationStandardOffsetUnits=m  TranslationROffset=0  TranslationROffsetUnits=m  TranslationThetaOffset=0  TranslationThetaOffsetUnits=deg  TranslationZOffset=0  TranslationZOffsetUnits=m
  F : PMIOPort  Side=Left
  F2 : PMIOPort  Port=2  Side=Right
  F1 : PMIOPort  Port=3  Side=Right
  connections:
  Inertia/RConn1 -- InertiaOriginTransform/RConn1
  ReferenceFrame/RConn1 -- InertiaOriginTransform/LConn1 -- base_link_base_fixed_joint_OriginTransform/LConn1 -- base_link_base_link_inertia_OriginTransform/LConn1 -- F/RConn1
  base_link_base_fixed_joint_OriginTransform/RConn1 -- F1/RConn1
  base_link_base_link_inertia_OriginTransform/RConn1 -- F2/RConn1

== system ur5_mb1/Subsystem/base_link_inertia ==
  Inertia : sm_lib/Body Elements/Inertia  InertiaType=Custom  Mass=4  MassUnits=kg  CenterOfMass=[0, 0, 0]  CenterOfMassUnits=m  MomentsOfInertia=[0.00443333156, 0.00443333156, 0.0072]  MomentsOfInertiaUnits=kg*m^2  ProductsOfInertia=[0, 0, 0]  ProductsOfInertiaUnits=kg*m^2  GraphicType=None  MarkerShape=Inertia  MarkerSize=20  GraphicVisPropType=SimpleVisualProperties  GraphicDiffuseColor=[0.5 0.5 0.5]  GraphicOpacity=1  GraphicSpecularColor=[0.5 0.5 0.5 1.0]  GraphicAmbientColor=[0.15 0.15 0.15 1.0]  GraphicEmissiveColor=[0.0 0.0 0.0 1.0]  GraphicShininess=75
  InertiaOriginTransform : sm_lib/Frames and Transforms/Rigid Transform  RotationMethod=RotationSequence  FollAlignAxisA=+X  BaseAlignAxisA=+Y  FollAlignAxisB=+Y  BaseAlignAxisB=+Z  RotationStandardAxis=+Z  RotationAngle=0  RotationAngleUnits=deg  RotationArbitraryAxis=[0 0 1]  RotationSequenceAxes=BaseAxes  RotationSequence=XYZ  RotationSequenceAngles=[0, 0, 0]  RotationSequenceAnglesUnits=rad  RotationMatrix=[1 0 0;0 1 0;0 0 1]  Quaternion=[1 0 0 0]  TranslationMethod=Cartesian  TranslationCartesianOffset=[0, 0, 0]  TranslationCartesianOffsetUnits=m  TranslationStandardAxis=+Z  TranslationStandardOffset=0  TranslationStandardOffsetUnits=m  TranslationROffset=0  TranslationROffsetUnits=m  TranslationThetaOffset=0  TranslationThetaOffsetUnits=deg  TranslationZOffset=0  TranslationZOffsetUnits=m
  ReferenceFrame : sm_lib/Frames and Transforms/Reference Frame
  Visual : sm_lib/Body Elements/File Solid  ExtGeomFileName=D:\WORK\school\cls\movepartom\ur\ur5_meshes\collision\base.stl  UnitType=Custom  ExtGeomFileUnits=m  StepReaderType=HEX  ExportConvexHullGeometry=off  InertiaType=Custom  BasedOnType=DensityFromFile  Density=1000  DensityUnits=kg/m^3  Mass=0  MassUnits=kg  CenterOfMass=[0, 0, 0]  CenterOfMassUnits=m  MomentsOfInertia=[0, 0, 0]  MomentsOfInertiaUnits=kg*m^2  ProductsOfInertia=[0, 0, 0]  ProductsOfInertiaUnits=kg*m^2  GraphicType=FromGeometry  MarkerShape=Sphere  MarkerSize=10  GraphicVisPropType=SimpleVisualProperties  GraphicDiffuseColor=[0.1,0.8,0.9]  GraphicOpacity=1  GraphicSpecularColor=[0.5 0.5 0.5 1.0]  GraphicAmbientColor=[0.15 0.15 0.15 1.0]  GraphicEmissiveColor=[0.0 0.0 0.0 1.0]  GraphicShininess=75  DoExposeReferenceFrame=on  SerializedFrames=<Frames/>
  VisualOriginTransform : sm_lib/Frames and Transforms/Rigid Transform  RotationMethod=RotationSequence  FollAlignAxisA=+X  BaseAlignAxisA=+Y  FollAlignAxisB=+Y  BaseAlignAxisB=+Z  RotationStandardAxis=+Z  RotationAngle=0  RotationAngleUnits=deg  RotationArbitraryAxis=[0 0 1]  RotationSequenceAxes=BaseAxes  RotationSequence=XYZ  RotationSequenceAngles=[0, 0, 3.141592653589793]  RotationSequenceAnglesUnits=rad  RotationMatrix=[1 0 0;0 1 0;0 0 1]  Quaternion=[1 0 0 0]  TranslationMethod=Cartesian  TranslationCartesianOffset=[0, 0, 0]  TranslationCartesianOffsetUnits=m  TranslationStandardAxis=+Z  TranslationStandardOffset=0  TranslationStandardOffsetUnits=m  TranslationROffset=0  TranslationROffsetUnits=m  TranslationThetaOffset=0  TranslationThetaOffsetUnits=deg  TranslationZOffset=0  TranslationZOffsetUnits=m
  shoulder_pan_joint_AxisTransform : sm_lib/Frames and Transforms/Rigid Transform  RotationMethod=ArbitraryAxis  FollAlignAxisA=+X  BaseAlignAxisA=+Y  FollAlignAxisB=+Y  BaseAlignAxisB=+Z  RotationStandardAxis=+Z  RotationAngle=0  RotationAngleUnits=rad  RotationArbitraryAxis=[1, 0, 0]  RotationSequenceAxes=FollowerAxes  RotationSequence=XYX  RotationSequenceAngles=[0 0 0]  RotationSequenceAnglesUnits=deg  RotationMatrix=[1 0 0;0 1 0;0 0 1]  Quaternion=[1 0 0 0]  TranslationMethod=Cartesian  TranslationCartesianOffset=[0, 0, 0]  TranslationCartesianOffsetUnits=m  TranslationStandardAxis=+Z  TranslationStandardOffset=0  TranslationStandardOffsetUnits=m  TranslationROffset=0  TranslationROffsetUnits=m  TranslationThetaOffset=0  TranslationThetaOffsetUnits=deg  TranslationZOffset=0  TranslationZOffsetUnits=m
  shoulder_pan_joint_OriginTransform : sm_lib/Frames and Transforms/Rigid Transform  RotationMethod=RotationSequence  FollAlignAxisA=+X  BaseAlignAxisA=+Y  FollAlignAxisB=+Y  BaseAlignAxisB=+Z  RotationStandardAxis=+Z  RotationAngle=0  RotationAngleUnits=deg  RotationArbitraryAxis=[0 0 1]  RotationSequenceAxes=BaseAxes  RotationSequence=XYZ  RotationSequenceAngles=[0, 0, 0]  RotationSequenceAnglesUnits=rad  RotationMatrix=[1 0 0;0 1 0;0 0 1]  Quaternion=[1 0 0 0]  TranslationMethod=Cartesian  TranslationCartesianOffset=[0, 0, 0.089159]  TranslationCartesianOffsetUnits=m  TranslationStandardAxis=+Z  TranslationStandardOffset=0  TranslationStandardOffsetUnits=m  TranslationROffset=0  TranslationROffsetUnits=m  TranslationThetaOffset=0  TranslationThetaOffsetUnits=deg  TranslationZOffset=0  TranslationZOffsetUnits=m
  F : PMIOPort  Side=Left
  F1 : PMIOPort  Port=2  Side=Right
  connections:
  Inertia/RConn1 -- InertiaOriginTransform/RConn1
  ReferenceFrame/RConn1 -- InertiaOriginTransform/LConn1 -- VisualOriginTransform/LConn1 -- shoulder_pan_joint_OriginTransform/LConn1 -- F/RConn1
  Visual/RConn1 -- VisualOriginTransform/RConn1
  shoulder_pan_joint_AxisTransform/RConn1 -- F1/RConn1
  shoulder_pan_joint_AxisTransform/LConn1 -- shoulder_pan_joint_OriginTransform/RConn1

== system ur5_mb1/Subsystem/flange ==
  Inertia : sm_lib/Body Elements/Inertia  InertiaType=Custom  Mass=0  MassUnits=kg  CenterOfMass=[0, 0, 0]  CenterOfMassUnits=m  MomentsOfInertia=[0, 0, 0]  MomentsOfInertiaUnits=kg*m^2  ProductsOfInertia=[0, 0, 0]  ProductsOfInertiaUnits=kg*m^2  GraphicType=None  MarkerShape=Inertia  MarkerSize=20  GraphicVisPropType=SimpleVisualProperties  GraphicDiffuseColor=[0.5 0.5 0.5]  GraphicOpacity=1  GraphicSpecularColor=[0.5 0.5 0.5 1.0]  GraphicAmbientColor=[0.15 0.15 0.15 1.0]  GraphicEmissiveColor=[0.0 0.0 0.0 1.0]  GraphicShininess=75
  InertiaOriginTransform : sm_lib/Frames and Transforms/Rigid Transform  RotationMethod=RotationSequence  FollAlignAxisA=+X  BaseAlignAxisA=+Y  FollAlignAxisB=+Y  BaseAlignAxisB=+Z  RotationStandardAxis=+Z  RotationAngle=0  RotationAngleUnits=deg  RotationArbitraryAxis=[0 0 1]  RotationSequenceAxes=BaseAxes  RotationSequence=XYZ  RotationSequenceAngles=[0, 0, 0]  RotationSequenceAnglesUnits=rad  RotationMatrix=[1 0 0;0 1 0;0 0 1]  Quaternion=[1 0 0 0]  TranslationMethod=Cartesian  TranslationCartesianOffset=[0, 0, 0]  TranslationCartesianOffsetUnits=m  TranslationStandardAxis=+Z  TranslationStandardOffset=0  TranslationStandardOffsetUnits=m  TranslationROffset=0  TranslationROffsetUnits=m  TranslationThetaOffset=0  TranslationThetaOffsetUnits=deg  TranslationZOffset=0  TranslationZOffsetUnits=m
  ReferenceFrame : sm_lib/Frames and Transforms/Reference Frame
  flange_tool0_OriginTransform : sm_lib/Frames and Transforms/Rigid Transform  RotationMethod=RotationSequence  FollAlignAxisA=+X  BaseAlignAxisA=+Y  FollAlignAxisB=+Y  BaseAlignAxisB=+Z  RotationStandardAxis=+Z  RotationAngle=0  RotationAngleUnits=deg  RotationArbitraryAxis=[0 0 1]  RotationSequenceAxes=BaseAxes  RotationSequence=XYZ  RotationSequenceAngles=[1.570796326794897, 0, 1.570796326794897]  RotationSequenceAnglesUnits=rad  RotationMatrix=[1 0 0;0 1 0;0 0 1]  Quaternion=[1 0 0 0]  TranslationMethod=Cartesian  TranslationCartesianOffset=[0, 0, 0]  TranslationCartesianOffsetUnits=m  TranslationStandardAxis=+Z  TranslationStandardOffset=0  TranslationStandardOffsetUnits=m  TranslationROffset=0  TranslationROffsetUnits=m  TranslationThetaOffset=0  TranslationThetaOffsetUnits=deg  TranslationZOffset=0  TranslationZOffsetUnits=m
  F : PMIOPort  Side=Left
  F1 : PMIOPort  Port=2  Side=Right
  connections:
  Inertia/RConn1 -- InertiaOriginTransform/RConn1
  ReferenceFrame/RConn1 -- InertiaOriginTransform/LConn1 -- flange_tool0_OriginTransform/LConn1 -- F/RConn1
  flange_tool0_OriginTransform/RConn1 -- F1/RConn1
